simulink model "L5"  (R2019b)
settings: Solver=FixedStepAuto  StartTime=0.0  StopTime=10.0  FixedStep=1e-4  RelTol=1e-3
InitFcn:
  | m = [1 1];      % масса звеньев
  | l = [1 1];      % длина звеньев
  | lc = [.5 .5];   % расст от СК звена до центра масс звена
  | I = [1 1];      % моменты инерции звеньев
  | Jm = [0 0];     % момент инерции редукторов?
  | r = [1 1];      % передаточные числа редукторов
  | D = [.1 .1];    % агрегированные коэффициенты демпфирования
  | 
  | g = 9.81;       % ускорение свободного падения
  | 
  | 
  | global rho;
  | rho = [
  |     m(1)*lc(1)^2 + m(2)*l(1)^2 + 2*m(2)*l(1)*lc(2)^2 + I(1),... % rho_1
  |     m(2)*lc(2)^2 + I(2),...                                     % rho_2
  |     m(2)*l(1)*lc(2),...                                         % rho_3
  |     r(1)^2*Jm(1),...                                            % rho_4
  |     r(2)^2*Jm(2),...                                            % rho_5
  |     (m(1)*lc(1) + m(2)*l(1))*g,...                              % rho_6
  |     m(2)*lc(2)*g,...                                            % rho_7
  |     m(2)*lc(2),...                                              % rho_8
  |     r(1)^2*D(1),...                                             % rho_9
  |     r(2)^2*D(2)                                                 % rho_10
  |     ];
  | 
  | 
  | % матрица вязкого трения
  | F = [
  |     rho(9) 0;
  |     0 rho(10)
  |     ];
  | 
  | A_ref = [1 1];      % амплитуды
  | psi_ref = [0 0];    % фазы
  | omega_ref = [1 2];  % частоты
  | 
  | w_ref_0 = [
  |     A_ref(1)*sin(psi_ref(1)),...
  |     omega_ref(1)*A_ref(1)*cos(psi_ref(1)),...
  |     A_ref(2)*sin(psi_ref(2)),...
  |     omega_ref(2)*A_ref(2)*cos(psi_ref(2))
  |     ];
  | 
  | Sref1 = [
  |     0 1;
  |     -omega_ref(1)^2 0
  |     ];
  | Sref2 = [
  |     0 1;
  |     -omega_ref(2)^2 0
  |     ];
  | 
  | Sref = blkdiag(Sref1, Sref2);
  | 
  | H_ref_p1 = [1 0];
  | H_ref_p2 = [1 0];
  | H_ref_p = blkdiag(H_ref_p1, H_ref_p2);
  | 
  | H_ref_v1 = [0 1];
  | H_ref_v2 = [0 1];
  | H_ref_v = blkdiag(H_ref_v1, H_ref_v2);
  | 
  | H_ref_a1 = [-omega_ref(1)^2 0];
  | H_ref_a2 = [-omega_ref(2)^2 0];
  | H_ref_a = blkdiag(H_ref_a1, H_ref_a2);
  | 
  | k_p = [100 100];
  | K_p = diag(k_p);
  | 
  | k_d = [100 100];
  | K_d = diag(k_d);
  | 
  | kappa = 1000;
  | 
  | A1 = [
  |     10 1;
  |     1 10
  |     ];
  | A2 = [
  |     20 2;
  |     2 20
  |     ];
  | 
  | A = [
  |     -A2 eye(size(A2));
  |     -A1 zeros(size(A1))
  |     ];
  | 
  | % остальные матрицы зависят от q и объявлены функциями
model workspace (MATLAB code in the model file):
  | m = [1 1];      % ����� �������
  | l = [1 1];      % ����� �������
  | lc = [.5 .5];   % ����� �� �� ����� �� ������ ���� �����
  | I = [1 1];      % ������� ������� �������
  | Jm = [0 0];        % ������ ������� ����������?
  | r = [1 1];      % ������������ ����� ����������
  | D = [.1 .1];    % �������������� ������������ �������������
  | 
  | g = 9.81;       % ��������� ���������� �������
  | 
  | 
  | rho = [
  |     m(1)*lc(1)^2 + m(2)*l(1)^2 + 2*m(2)*l(1)*lc(2)^2 + I(1),... % rho_1
  |     m(2)*lc(2)^2 + I(2),...                                     % rho_2
  |     m(2)*l(1)*lc(2),...                                         % rho_3
  |     r(1)^2*Jm(1),...                                            % rho_4
  |     r(2)^2*Jm(2),...                                            % rho_5
  |     (m(1)*lc(1) + m(2)*l(1))*g,...                              % rho_6
  |     m(2)*lc(2)*g,...                                            % rho_7
  |     m(2)*lc(2),...                                              % rho_8
  |     r(1)^2*D(1),...                                             % rho_9
  |     r(2)^2*D(2)                                                 % rho_10
  |     ];
  | 
  | 
  | % ������� ������� ������
  | F = [
  |     rho(9) 0;
  |     0 rho(10)
  |     ];
  | 
  | A_ref = [1 1];      % ���������
  | psi_ref = [0 0];    % ����
  | omega_ref = [1 2];  % �������
  | 
  | w_ref_0 = [
  |     A_ref(1)*sin(psi_ref(1)),...
  |     omega_ref(1)*A_ref(1)*cos(psi_ref(1)),...
  |     A_ref(2)*sin(psi_ref(2)),...
  |     omega_ref(2)*A_ref(2)*cos(psi_ref(2))
  |     ];
  | 
  | Sref1 = [
  |     0 1;
  |     -omega_ref(1)^2 0
  |     ];
  | Sref2 = [
  |     0 1;
  |     -omega_ref(1)^2 0
  |     ];
  | 
  | Sref = blkdiag(Sref1, Sref2);
  | 
  | H_ref_p1 = [1 0];
  | H_ref_p2 = [1 0];
  | H_ref_p = blkdiag(H_ref_p1, H_ref_p2);
  | 
  | H_ref_v1 = [0 1];
  | H_ref_v2 = [0 1];
  | H_ref_v = blkdiag(H_ref_v1, H_ref_v2);
  | 
  | H_ref_a1 = [-omega_ref(1)^2 0];
  | H_ref_a2 = [-omega_ref(2)^2 0];
  | H_ref_a = blkdiag(H_ref_a1, H_ref_a2);
  | 
  | % ��������� ������� ������� �� q � ��������� ���������
  | function M = moments(q)
  |     c2 = cos(q(2));
  |     M = [
  |         rho(1) + rho(2) + 2*rho(3)*c2 + rho(4), rho(2) + rho(3)*c2;
  |         rho(2) + rho(3)*c2, rho(2) + rho(5);
  |         ];
  | end
  | 
  | function C = coreolis(dq, q)
  |     s2 = sin(q(2));
  |     C = [
  |         -rho(3)*s2*dq(2), -rho(3)*s2*(dq(1) + dq(2));
  |         rho(3)*s2*dq(1), 0
  |         ];
  | end
  | 
  | function G = gravitational(q)
  |     c1 = cos(q(1));
  |     c12 = cos(q(1) + q(2));
  |     G = [
  |         rho(6)*c1 + rho(7)*c12,...
  |         rho(8)*c12
  |         ];
  | end
settings Model: OrderedModelArguments=off  Creator=bedla  LastModifiedBy=bedla

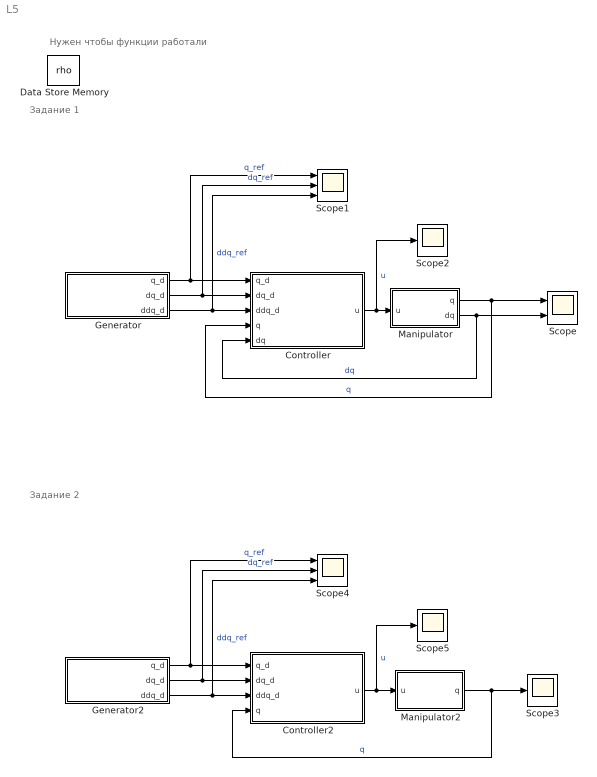
== system L5 ==
  note: Задание 1
  note: Нужен чтобы функции работали
  note: Задание 2
  Controller : Subsystem
  Controller2 : Subsystem
  Data Store Memory : DataStoreMemory  DataStoreName=rho  ReadBeforeWriteMsg=warning  WriteAfterWriteMsg=warning  WriteAfterReadMsg=warning  InitialValue=rho  ShowAdditionalParam=off  OutDataTypeStr=double
  Generator : Subsystem
  Generator2 : Subsystem
  Manipulator : Subsystem
  Manipulator2 : Subsystem
  Scope : Scope  NumInputPorts=2
  Scope1 : Scope  NumInputPorts=3
  Scope2 : Scope
  Scope3 : Scope
  Scope4 : Scope  NumInputPorts=3
  Scope5 : Scope
  wires:
  Controller/1(u) -> Scope2/1, Manipulator/1(u)  "u"
  Manipulator/1(q) -> Controller/4(q), Scope/1  "q"
  Manipulator/2(dq) -> Controller/5(dq), Scope/2  "dq"
  Generator/1(q_d) -> Scope1/1, Controller/1(q_d)  "q_ref"
  Generator/2(dq_d) -> Scope1/2, Controller/2(dq_d)  "dq_ref"
  Generator/3(ddq_d) -> Scope1/3, Controller/3(ddq_d)  "ddq_ref"
  Generator2/3(ddq_d) -> Scope4/3, Controller2/3(ddq_d)  "ddq_ref"
  Generator2/2(dq_d) -> Scope4/2, Controller2/2(dq_d)  "dq_ref"
  Controller2/1(u) -> Manipulator2/1(u), Scope5/1  "u"
  Manipulator2/1(q) -> Controller2/4(q), Scope3/1  "q"
  Generator2/1(q_d) -> Scope4/1, Controller2/1(q_d)  "q_ref"

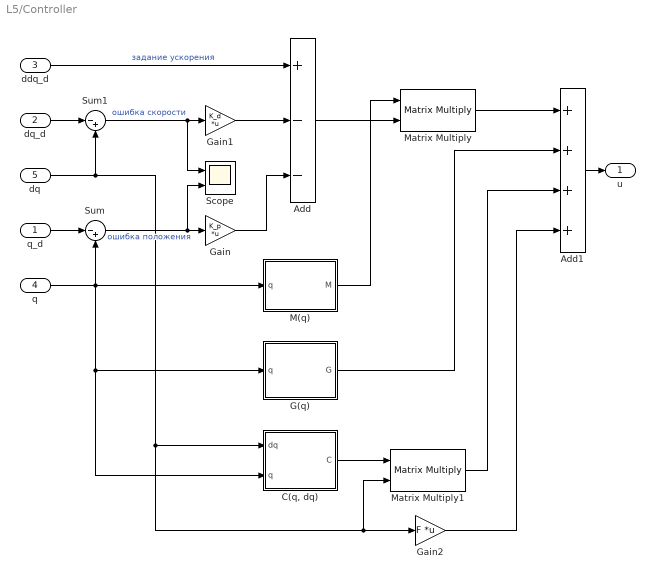
== system L5/Controller ==
  q_d : Inport
  dq_d : Inport  Port=2
  ddq_d : Inport  Port=3
  q : Inport  Port=4
  dq : Inport  Port=5
  Add : Sum  Inputs=+--
  Add1 : Sum  Inputs=++++
  "C(q, dq)" : MATLAB Function
  G(q) : MATLAB Function  TreatAsAtomicUnit=on
  Gain : Gain  Gain=K_p  Multiplication=Matrix(K*u) (u vector)
  Gain1 : Gain  Gain=K_d  Multiplication=Matrix(K*u) (u vector)
  Gain2 : Gain  Gain=F  Multiplication=Matrix(K*u) (u vector)
  M(q) : MATLAB Function  TreatAsAtomicUnit=on
  Matrix Multiply : Product  Multiplication=Matrix(*)
  Matrix Multiply1 : Product  Multiplication=Matrix(*)
  Scope : Scope  NumInputPorts=2
  Sum : Sum  Inputs=|-+
  Sum1 : Sum  Inputs=|-+
  u : Outport
  wires:
  q_d/1 -> Sum/1
  q/1 -> "C(q, dq)"/2(q), G(q)/1(q), M(q)/1(q), Sum/2
  Sum/1 -> Scope/2, Gain/1  "ошибка положения"
  dq_d/1 -> Sum1/1
  dq/1 -> Matrix Multiply1/2, Gain2/1, "C(q, dq)"/1(dq), Sum1/2
  Sum1/1 -> Scope/1, Gain1/1  "ошибка скорости"
  Gain/1 -> Add/3
  Gain1/1 -> Add/2
  ddq_d/1 -> Add/1  "задание ускорения"
  Add/1 -> Matrix Multiply/2
  M(q)/1(M) -> Matrix Multiply/1
  "C(q, dq)"/1(C) -> Matrix Multiply1/1
  Matrix Multiply/1 -> Add1/1
  G(q)/1(G) -> Add1/2
  Gain2/1 -> Add1/4
  Matrix Multiply1/1 -> Add1/3
  Add1/1 -> u/1

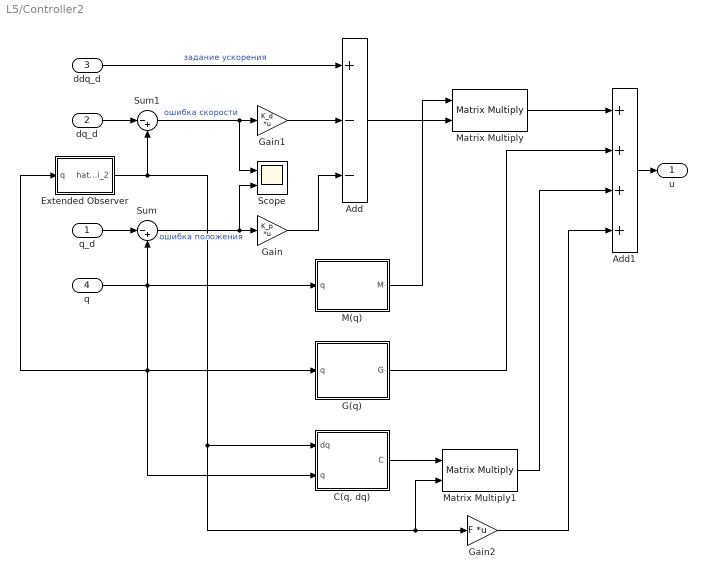
== system L5/Controller2 ==
  q_d : Inport
  dq_d : Inport  Port=2
  ddq_d : Inport  Port=3
  q : Inport  Port=4
  Add : Sum  Inputs=+--
  Add1 : Sum  Inputs=++++
  "C(q, dq)" : MATLAB Function
  Extended Observer : Subsystem
  G(q) : MATLAB Function  TreatAsAtomicUnit=on
  Gain : Gain  Gain=K_p  Multiplication=Matrix(K*u) (u vector)
  Gain1 : Gain  Gain=K_d  Multiplication=Matrix(K*u) (u vector)
  Gain2 : Gain  Gain=F  Multiplication=Matrix(K*u) (u vector)
  M(q) : MATLAB Function  TreatAsAtomicUnit=on
  Matrix Multiply : Product  Multiplication=Matrix(*)
  Matrix Multiply1 : Product  Multiplication=Matrix(*)
  Scope : Scope  NumInputPorts=2
  Sum : Sum  Inputs=|-+
  Sum1 : Sum  Inputs=|-+
  u : Outport
  wires:
  q_d/1 -> Sum/1
  q/1 -> Extended Observer/1(q), "C(q, dq)"/2(q), G(q)/1(q), M(q)/1(q), Sum/2
  Sum/1 -> Scope/2, Gain/1  "ошибка положения"
  dq_d/1 -> Sum1/1
  Extended Observer/1(hat xi_2) -> Matrix Multiply1/2, Gain2/1, "C(q, dq)"/1(dq), Sum1/2
  Sum1/1 -> Scope/1, Gain1/1  "ошибка скорости"
  Gain/1 -> Add/3
  Gain1/1 -> Add/2
  ddq_d/1 -> Add/1  "задание ускорения"
  Add/1 -> Matrix Multiply/2
  M(q)/1(M) -> Matrix Multiply/1
  "C(q, dq)"/1(C) -> Matrix Multiply1/1
  Matrix Multiply/1 -> Add1/1
  G(q)/1(G) -> Add1/2
  Gain2/1 -> Add1/4
  Matrix Multiply1/1 -> Add1/3
  Add1/1 -> u/1

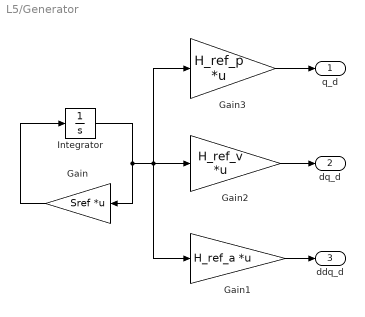
== system L5/Generator ==
  Gain : Gain  Gain=Sref  Multiplication=Matrix(K*u) (u vector)
  Gain1 : Gain  Gain=H_ref_a  Multiplication=Matrix(K*u) (u vector)
  Gain2 : Gain  Gain=H_ref_v  Multiplication=Matrix(K*u) (u vector)
  Gain3 : Gain  Gain=H_ref_p  Multiplication=Matrix(K*u) (u vector)
  Integrator : Integrator  InitialCondition=w_ref_0
  q_d : Outport
  dq_d : Outport  Port=2
  ddq_d : Outport  Port=3
  wires:
  Gain/1 -> Integrator/1
  Integrator/1 -> Gain/1, Gain3/1, Gain2/1, Gain1/1
  Gain1/1 -> ddq_d/1
  Gain2/1 -> dq_d/1
  Gain3/1 -> q_d/1

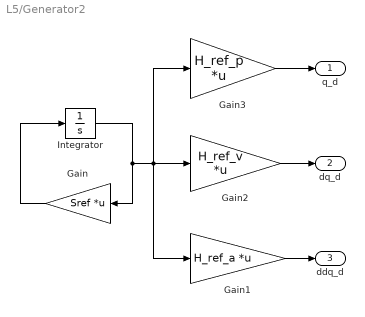
== system L5/Generator2 ==
  Gain : Gain  Gain=Sref  Multiplication=Matrix(K*u) (u vector)
  Gain1 : Gain  Gain=H_ref_a  Multiplication=Matrix(K*u) (u vector)
  Gain2 : Gain  Gain=H_ref_v  Multiplication=Matrix(K*u) (u vector)
  Gain3 : Gain  Gain=H_ref_p  Multiplication=Matrix(K*u) (u vector)
  Integrator : Integrator  InitialCondition=w_ref_0
  q_d : Outport
  dq_d : Outport  Port=2
  ddq_d : Outport  Port=3
  wires:
  Gain/1 -> Integrator/1
  Integrator/1 -> Gain/1, Gain3/1, Gain2/1, Gain1/1
  Gain1/1 -> ddq_d/1
  Gain2/1 -> dq_d/1
  Gain3/1 -> q_d/1

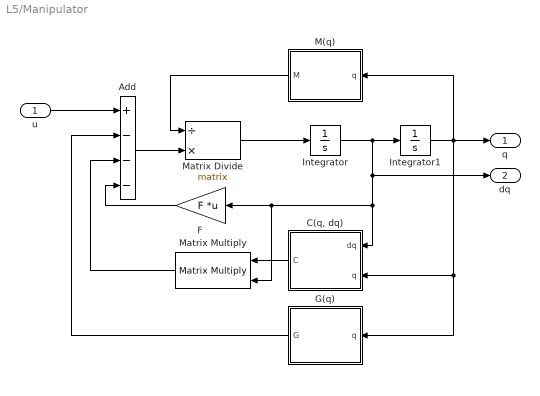
== system L5/Manipulator ==
  u : Inport
  Add : Sum  Inputs=+---
  "C(q, dq)" : MATLAB Function
  F : Gain  Gain=F  Multiplication=Matrix(K*u) (u vector)
  G(q) : MATLAB Function  TreatAsAtomicUnit=on
  Integrator : Integrator
  Integrator1 : Integrator
  M(q) : MATLAB Function  TreatAsAtomicUnit=on
  Matrix Divide : Product  Inputs=/*  Multiplication=Matrix(*)
  Matrix Multiply : Product  Multiplication=Matrix(*)
  q : Outport
  dq : Outport  Port=2
  wires:
  Matrix Divide/1 -> Integrator/1
  Add/1 -> Matrix Divide/2
  Integrator/1 -> dq/1, "C(q, dq)"/1(dq), Matrix Multiply/2, F/1, Integrator1/1
  Matrix Multiply/1 -> Add/3
  Integrator1/1 -> q/1, M(q)/1(q), G(q)/1(q), "C(q, dq)"/2(q)
  M(q)/1(M) -> Matrix Divide/1
  u/1 -> Add/1
  G(q)/1(G) -> Add/2
  "C(q, dq)"/1(C) -> Matrix Multiply/1
  F/1 -> Add/4

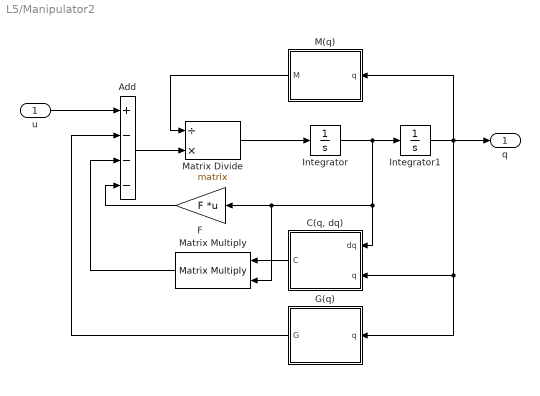
== system L5/Manipulator2 ==
  u : Inport
  Add : Sum  Inputs=+---
  "C(q, dq)" : MATLAB Function
  F : Gain  Gain=F  Multiplication=Matrix(K*u) (u vector)
  G(q) : MATLAB Function  TreatAsAtomicUnit=on
  Integrator : Integrator
  Integrator1 : Integrator
  M(q) : MATLAB Function  TreatAsAtomicUnit=on
  Matrix Divide : Product  Inputs=/*  Multiplication=Matrix(*)
  Matrix Multiply : Product  Multiplication=Matrix(*)
  q : Outport
  wires:
  Matrix Divide/1 -> Integrator/1
  Add/1 -> Matrix Divide/2
  Integrator/1 -> "C(q, dq)"/1(dq), Matrix Multiply/2, F/1, Integrator1/1
  Matrix Multiply/1 -> Add/3
  Integrator1/1 -> q/1, M(q)/1(q), G(q)/1(q), "C(q, dq)"/2(q)
  M(q)/1(M) -> Matrix Divide/1
  u/1 -> Add/1
  G(q)/1(G) -> Add/2
  "C(q, dq)"/1(C) -> Matrix Multiply/1
  F/1 -> Add/4

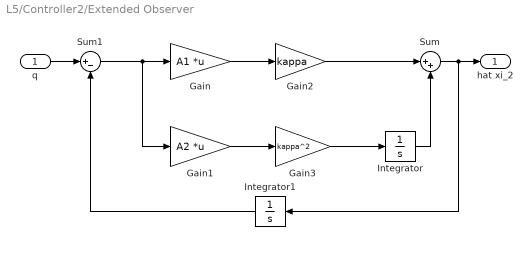
== system L5/Controller2/Extended Observer ==
  q : Inport
  Gain : Gain  Gain=A1  Multiplication=Matrix(K*u) (u vector)
  Gain1 : Gain  Gain=A2  Multiplication=Matrix(K*u) (u vector)
  Gain2 : Gain  Gain=kappa
  Gain3 : Gain  Gain=kappa^2
  Integrator : Integrator
  Integrator1 : Integrator
  Sum : Sum  Inputs=|++
  Sum1 : Sum  Inputs=|+-
  hat xi_2 : Outport
  wires:
  Gain1/1 -> Gain3/1
  Gain/1 -> Gain2/1
  Gain3/1 -> Integrator/1
  Gain2/1 -> Sum/1
  Integrator/1 -> Sum/2
  Sum/1 -> Integrator1/1, hat xi_2/1
  q/1 -> Sum1/1
  Sum1/1 -> Gain1/1, Gain/1
  Integrator1/1 -> Sum1/2

== matlab function L5/Manipulator/C(q, dq) ==
  settings: updateMethod=DISCRETE
  data: dq input; q input; C output; rho data_store_memory
function C = coreolis(dq, q)
    global rho;
    s2 = sin(q(2));
    C = [
        -rho(3)*s2*dq(2) -rho(3)*s2*(dq(1) + dq(2));
        rho(3)*s2*dq(1) 0
        ];
end

== matlab function L5/Manipulator/M(q) ==
  settings: updateMethod=DISCRETE
  data: q input; M output; rho data_store_memory
function M = moments(q)
    global rho;
    c2 = cos(q(2));
    M = [
        rho(1) + rho(2) + 2*rho(3)*c2 + rho(4), rho(2) + rho(3)*c2;
        rho(2) + rho(3)*c2, rho(2) + rho(5);
        ];
end

== matlab function L5/Manipulator/G(q) ==
  settings: updateMethod=DISCRETE
  data: q input; G output; rho data_store_memory
function G = gravit(q)
    global rho;
    c1 = cos(q(1));
    c12 = cos(q(1) + q(2));
    G = [
        rho(6)*c1 + rho(7)*c12;
        rho(8)*c12
        ];
end

== matlab function L5/Controller/C(q, dq) ==
  settings: updateMethod=DISCRETE
  data: dq input; q input; C output; rho data_store_memory
function C = coreolis(dq, q)
    global rho;
    s2 = sin(q(2));
    C = [
        -rho(3)*s2*dq(2) -rho(3)*s2*(dq(1) + dq(2));
        rho(3)*s2*dq(1) 0
        ];
end

== matlab function L5/Controller/G(q) ==
  settings: updateMethod=DISCRETE
  data: q input; G output; rho data_store_memory
function G = gravit(q)
    global rho;
    c1 = cos(q(1));
    c12 = cos(q(1) + q(2));
    G = [
        rho(6)*c1 + rho(7)*c12;
        rho(8)*c12
        ];
end

== matlab function L5/Controller/M(q) ==
  settings: updateMethod=DISCRETE
  data: q input; M output; rho data_store_memory
function M = moments(q)
    global rho;
    c2 = cos(q(2));
    M = [
        rho(1) + rho(2) + 2*rho(3)*c2 + rho(4) rho(2) + rho(3)*c2;
        rho(2) + rho(3)*c2 rho(2) + rho(5);
        ];
end

== matlab function L5/Controller2/C(q, dq) ==
  settings: updateMethod=DISCRETE
  data: dq input; q input; C output; rho data_store_memory
function C = coreolis(dq, q)
    global rho;
    s2 = sin(q(2));
    C = [
        -rho(3)*s2*dq(2) -rho(3)*s2*(dq(1) + dq(2));
        rho(3)*s2*dq(1) 0
        ];
end

== matlab function L5/Controller2/G(q) ==
  settings: updateMethod=DISCRETE
  data: q input; G output; rho data_store_memory
function G = gravit(q)
    global rho;
    c1 = cos(q(1));
    c12 = cos(q(1) + q(2));
    G = [
        rho(6)*c1 + rho(7)*c12;
        rho(8)*c12
        ];
end

== matlab function L5/Controller2/M(q) ==
  settings: updateMethod=DISCRETE
  data: q input; M output; rho data_store_memory
function M = moments(q)
    global rho;
    c2 = cos(q(2));
    M = [
        rho(1) + rho(2) + 2*rho(3)*c2 + rho(4) rho(2) + rho(3)*c2;
        rho(2) + rho(3)*c2 rho(2) + rho(5);
        ];
end

== matlab function L5/Manipulator2/C(q, dq) ==
  settings: updateMethod=DISCRETE
  data: dq input; q input; C output; rho data_store_memory
function C = coreolis(dq, q)
    global rho;
    s2 = sin(q(2));
    C = [
        -rho(3)*s2*dq(2) -rho(3)*s2*(dq(1) + dq(2));
        rho(3)*s2*dq(1) 0
        ];
end

== matlab function L5/Manipulator2/G(q) ==
  settings: updateMethod=DISCRETE
  data: q input; G output; rho data_store_memory
function G = gravit(q)
    global rho;
    c1 = cos(q(1));
    c12 = cos(q(1) + q(2));
    G = [
        rho(6)*c1 + rho(7)*c12;
        rho(8)*c12
        ];
end

== matlab function L5/Manipulator2/M(q) ==
  settings: updateMethod=DISCRETE
  data: q input; M output; rho data_store_memory
function M = moments(q)
    global rho;
    c2 = cos(q(2));
    M = [
        rho(1) + rho(2) + 2*rho(3)*c2 + rho(4), rho(2) + rho(3)*c2;
        rho(2) + rho(3)*c2, rho(2) + rho(5);
        ];
end
